simulink model "EE160_Lab_4"  (R2024b)
settings: Solver=VariableStepAuto  StartTime=0.0  StopTime=1  RelTol=1e-3
undefined symbols (not defined in the file or in its folder): Angle, Magnitude
libraries: spsCurrentMeasurementLib x3, spsLinearTransformerLib x2, spsSeriesRLCBranchLib x2, spsVoltageMeasurementLib x2, spsACVoltageSourceLib x1, sps_lib x1
settings Model: Creator=dhair  LastModifiedBy=Bhavya Prajapati

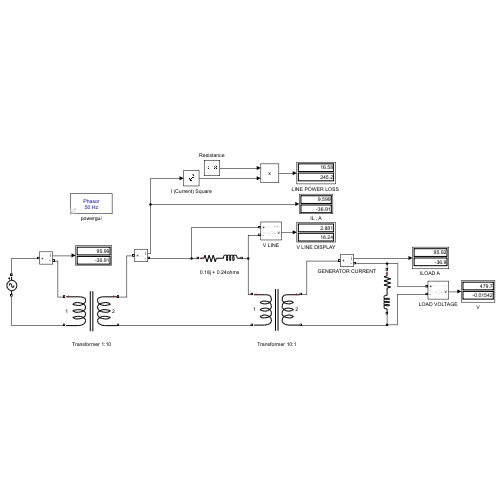
[thumbnail: Simulink's stored preview of the top-level diagram]
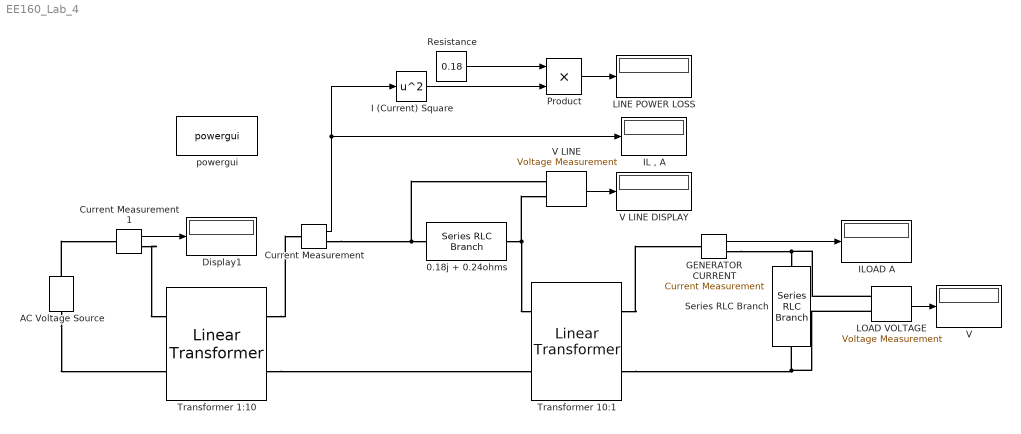
== system EE160_Lab_4 ==
  " Transformer 10:1" : spsLinearTransformerLib/Linear Transformer  UNITS=SI  NominalPower=[ 250e6 60 ]  winding1="[4800  0.000001  0.000001]"  winding2="[480  0.000001  0.000001]"  ThreeWindings=off  winding3=[3.15e+05 0.7938 0.084225]  RmLm=[1.0804e+06 2866]  Measurements=None  DataType=on
  " Transformer 1:10" : spsLinearTransformerLib/Linear Transformer  UNITS=SI  NominalPower=[ 250e6 60 ]  winding1="[480  0.000001  0.000001]"  winding2="[4800  0.000001  0.000001]"  ThreeWindings=off  winding3=[3.15e+05 0.7938 0.084225]  RmLm=[1.0804e+06 2866]  Measurements=None  DataType=on
  0.18j + 0.24ohms : spsSeriesRLCBranchLib/Series RLC Branch  LConnTagsString=__new0  RConnTagsString=__new0  BranchType=RL  Resistance=0.18  Inductance=0.0007643312  SetiL0=off  InitialCurrent=0  Capacitance=1e-6  Setx0=off  InitialVoltage=0  Measurements=None
  AC Voltage Source : spsACVoltageSourceLib/AC Voltage Source  Amplitude=480  Phase=0  Frequency=50  SampleTime=1  Measurements=None  BusType=swing  Pref=10e3  Qref=0  Qmin=-inf  Qmax=+inf
  Current Measurement : spsCurrentMeasurementLib/Current Measurement  PhasorSimulation=on  OutputType=Magnitude-Angle  PSBequivalent=0
  Current Measurement1 : spsCurrentMeasurementLib/Current Measurement  PhasorSimulation=on  OutputType=Magnitude-Angle  PSBequivalent=0
  Display1 : Display
  GENERATOR CURRENT : spsCurrentMeasurementLib/Current Measurement  PhasorSimulation=on  OutputType=Magnitude-Angle  PSBequivalent=0
  I (Current) Square : Math  Operator=square
  "IL , A" : Display
  "ILOAD A " : Display
  "LINE POWER LOSS " : Display
  LOAD VOLTAGE : spsVoltageMeasurementLib/Voltage Measurement  PhasorSimulation=on  OutputType=Magnitude-Angle  PSBequivalent=0
  Product : Product
  Resistance : Constant  Value=0.18
  Series RLC Branch : spsSeriesRLCBranchLib/Series RLC Branch  LConnTagsString=__new0  RConnTagsString=__new0  BranchType=RL  Resistance=4  Inductance=0.0095541401  SetiL0=off  InitialCurrent=0  Capacitance=1e-6  Setx0=off  InitialVoltage=0  Measurements=None
  V : Display
  V LINE : spsVoltageMeasurementLib/Voltage Measurement  PhasorSimulation=on  OutputType=Magnitude-Angle  PSBequivalent=0
  V LINE DISPLAY : Display
  powergui : sps_lib/powergui  Priority=1  SimulationMode=Phasor  SampleTime=50e-6  frequency=50  Iterations=50  frequencyindice=50  Pbase=100e6  ErrMax=1e-4  UnitsV=kV  UnitsW=MW  buscounter=0  FunctionMessages=off  echomessages=off  EnableUseOfTLC=off  CurrentSourceSwitches=off  DisableSnubberDevices=off  DisableRonSwitches=off  DisableVfSwitches=off  DisplayEquations=off  AutomaticDiscreteSolvers=off  SolverType=Tustin/Backward Euler (TBE)  Interpol=off  ExternalGateDelay=off  methode=off  Ts=100  x0status=blocks  SPID=on  SwTol=0  HookPort=off  NonlinearTolerance=1e-4  nMaxIteration=100  ContinueOnMaxIteration=off  RestoreLinks=warning  ResistiveCurrentMeasurement=off  Frange=[0:2:500]  Ylog=off  Xlog=on  ShowGrid=off  save=off  variable=ZData  structure=0  ZoomFFT=off  StartTime=0.0  cycles=1  DisplayStyle=1  fundamental=60  FreqAxis=off  MaxFrequency=1000  frequencyindicesteady=1  RmsSteady=1  display=off
  wires:
  Current Measurement/1 -> I (Current) Square/1, "IL , A"/1
  Product/1 -> "LINE POWER LOSS "/1
  I (Current) Square/1 -> Product/2
  Resistance/1 -> Product/1
  LOAD VOLTAGE/1 -> V/1
  Current Measurement1/1 -> Display1/1
  GENERATOR CURRENT/1 -> "ILOAD A "/1
  V LINE/1 -> V LINE DISPLAY/1
  connections:
  Current Measurement/RConn1 -- V LINE/LConn1 -- 0.18j + 0.24ohms/LConn1
  LOAD VOLTAGE/LConn1 -- GENERATOR CURRENT/RConn1 -- Series RLC Branch/LConn1
  LOAD VOLTAGE/LConn2 -- " Transformer 10:1"/RConn2 -- Series RLC Branch/RConn1
  AC Voltage Source/LConn1 -- " Transformer 1:10"/LConn2
  " Transformer 1:10"/RConn1 -- Current Measurement/LConn1
  AC Voltage Source/RConn1 -- Current Measurement1/LConn1
  Current Measurement1/RConn1 -- " Transformer 1:10"/LConn1
  0.18j + 0.24ohms/RConn1 -- V LINE/LConn2 -- " Transformer 10:1"/LConn1
  " Transformer 1:10"/RConn2 -- " Transformer 10:1"/LConn2
  " Transformer 10:1"/RConn1 -- GENERATOR CURRENT/LConn1
